simulink model "SignalModelL4"  (R2017a)
settings: Solver=FixedStepAuto  StartTime=0.0  StopTime=10  FixedStep=0.01  RelTol=1e-3
values from neighbouring files (symbols this model uses):
  kd = 0.0842434289666    [matlab.mat]
  kd2 = 0.726167888094    [matlab.mat]
  ki = 0.0039872217887    [matlab.mat]
  ki2 = 1.30710219857    [matlab.mat]
  kp = 0.241923956026    [matlab.mat]
  kp2 = 0.344066439864    [matlab.mat]
libraries: checkpacklib x1
settings Model: Creator=roman  LastModifiedBy=roman

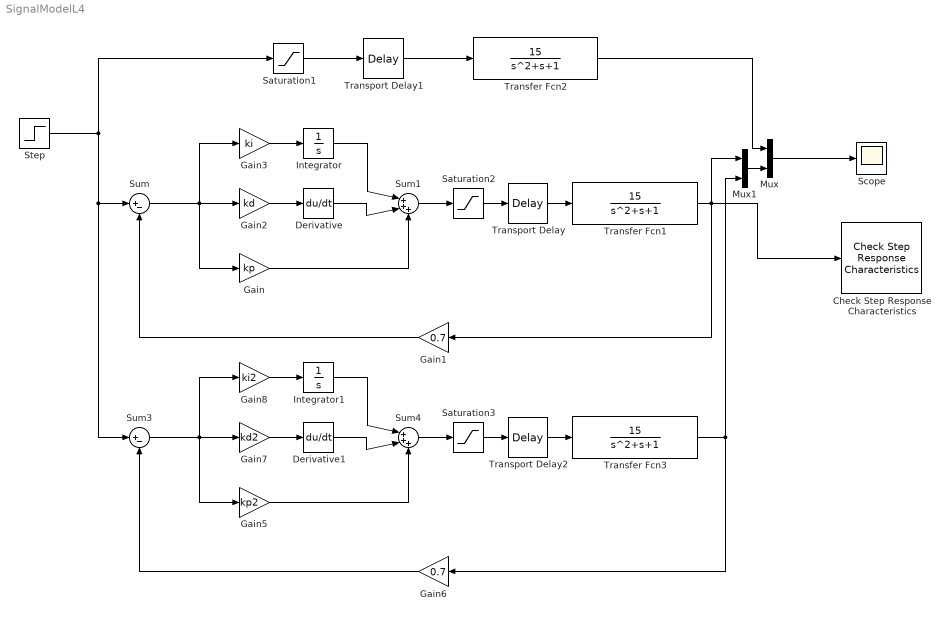
== system SignalModelL4 ==
  Check Step Response Characteristics : checkpacklib/Check Step Response  Characteristics  InstantiateOnLoad=on  enabled=on  stopWhenAssertionFail=off  export=off  ViewDlgPos=[100.333333333333 199.666666666667 510 390]  OpenViewOnLoad=off  LaunchViewOnOpen=off  TimeUnits=seconds  EnableStepResponseBound=on  InitialValue=0  FinalValue=1  StepTime=0  RiseTime=2  PercentRise=80  SettlingTime=6  PercentSettling=1  PercentOvershoot=10  PercentUndershoot=1
  Derivative : Derivative
  Derivative1 : Derivative
  Gain : Gain  Gain=kp
  Gain1 : Gain  Gain=0.7
  Gain2 : Gain  Gain=kd
  Gain3 : Gain  Gain=ki
  Gain5 : Gain  Gain=kp2
  Gain6 : Gain  Gain=0.7
  Gain7 : Gain  Gain=kd2
  Gain8 : Gain  Gain=ki2
  Integrator : Integrator
  Integrator1 : Integrator
  Mux : Mux  Inputs=2
  Mux1 : Mux  Inputs=2
  Saturation1 : Saturate  UpperLimit=2000  LowerLimit=-2000
  Saturation2 : Saturate  UpperLimit=2000  LowerLimit=-2000
  Saturation3 : Saturate  UpperLimit=2000  LowerLimit=-2000
  Scope : Scope
  Step : Step  Time=0  SampleTime=0
  Sum : Sum  Inputs=|+-
  Sum1 : Sum  Inputs=|+++
  Sum3 : Sum  Inputs=|+-
  Sum4 : Sum  Inputs=|+++
  Transfer Fcn1 : TransferFcn  Numerator=[15]  Denominator=[1 1 1]
  Transfer Fcn2 : TransferFcn  Numerator=[15]  Denominator=[1 1 1]
  Transfer Fcn3 : TransferFcn  Numerator=[15]  Denominator=[1 1 1]
  Transport Delay : TransportDelay  DelayTime=0.1
  Transport Delay1 : TransportDelay  DelayTime=0.1
  Transport Delay2 : TransportDelay  DelayTime=0.1
  wires:
  Transport Delay/1 -> Transfer Fcn1/1
  Transfer Fcn1/1 -> Mux1/1, Check Step Response Characteristics/1, Gain1/1
  Transport Delay1/1 -> Transfer Fcn2/1
  Mux/1 -> Scope/1
  Saturation2/1 -> Transport Delay/1
  Sum/1 -> Gain3/1, Gain/1, Gain2/1
  Gain1/1 -> Sum/2
  Gain3/1 -> Integrator/1
  Gain2/1 -> Derivative/1
  Gain/1 -> Sum1/3
  Derivative/1 -> Sum1/2
  Integrator/1 -> Sum1/1
  Sum1/1 -> Saturation2/1
  Saturation1/1 -> Transport Delay1/1
  Transfer Fcn2/1 -> Mux/1
  Gain8/1 -> Integrator1/1
  Gain5/1 -> Sum4/3
  Integrator1/1 -> Sum4/1
  Sum4/1 -> Saturation3/1
  Gain6/1 -> Sum3/2
  Derivative1/1 -> Sum4/2
  Sum3/1 -> Gain8/1, Gain5/1, Gain7/1
  Step/1 -> Saturation1/1, Sum3/1, Sum/1
  Saturation3/1 -> Transport Delay2/1
  Gain7/1 -> Derivative1/1
  Transport Delay2/1 -> Transfer Fcn3/1
  Mux1/1 -> Mux/2
  Transfer Fcn3/1 -> Mux1/2, Gain6/1
